simulink model "ieee80211n"  (Simulink 6.0)
settings: Solver=VariableStepDiscrete  StartTime=0.0  StopTime=inf  RelTol=1e-3
PreLoadFcn:
  | load IEEE80211n_init;
values from neighbouring files (symbols this model uses):
  params =     [IEEE80211n_init.mat]    (also in IEEE80211n_settings.m = p)
undefined symbols (not defined in the file or in its folder): magnitude
libraries: commblkintrlv2 x196, dspsigops x143, simulink x136, commdigbbndam2 x98, dspmtrx3 x96, dspsigattribs x69, dspstat3 x38, commutil2 x32, commsequence2 x26, commcnvcod2 x10, dspindex x9, dspmlti3 x8
(part 2 of 12)

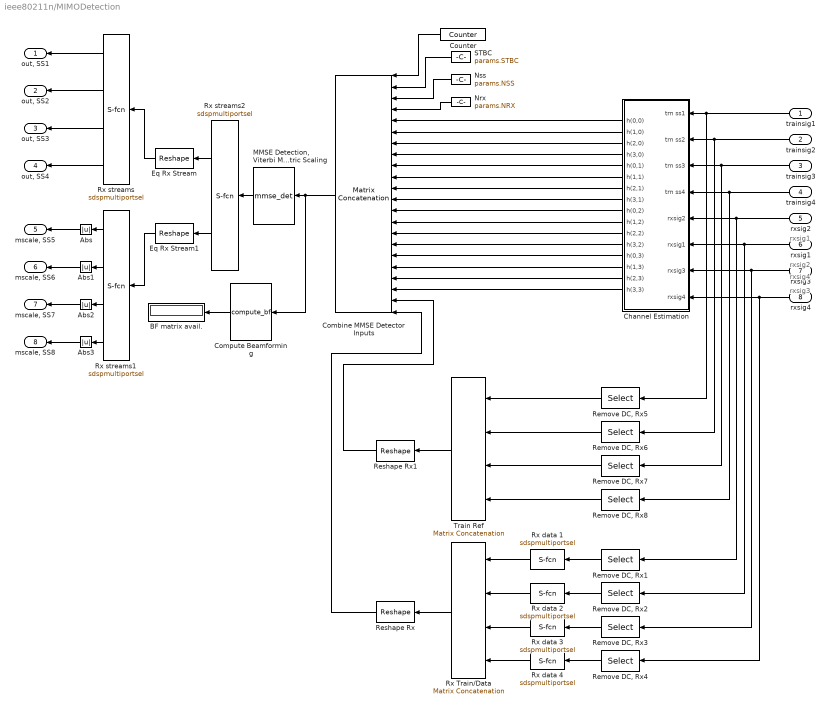
== system ieee80211n/MIMODetection ==
  note: rxsig1
  note: rxsig2
  note: rxsig3
  note: rxsig4
  trainsig1 : Inport  Orientation=left  Port=1  LatchInput=off
  trainsig2 : Inport  Orientation=left  Port=2  LatchInput=off
  trainsig3 : Inport  Orientation=left  Port=3  LatchInput=off
  trainsig4 : Inport  Orientation=left  Port=4  LatchInput=off
  rxsig2 : Inport  Orientation=left  Port=5  LatchInput=off
  rxsig1 : Inport  Orientation=left  Port=6  LatchInput=off
  rxsig3 : Inport  Orientation=left  Port=7  LatchInput=off
  rxsig4 : Inport  Orientation=left  Port=8  LatchInput=off
  Abs{,1..3} (4 alike) : Abs  Orientation=left
  BF matrix avail. : Display
  Channel Estimation : Subsystem  Orientation=left
  Combine MMSE Detector Inputs : simulink/Math Operations/Matrix Concatenation  Orientation=left  numInports=22  catMethod=Vertical
  Compute Beamforming : MATLABFcn  Orientation=left  MATLABFcn=compute_bf  OutputDimensions=[1 1]  Output1D=off
  Counter : dspswit3/Counter  Orientation=left  Direction=Up  CountEvent=Free running  CounterSize=32 bits  MaxCount=255  InitialCount=0  Output=Count  HitValue=32  ResetInput=off  SamplesPerFrame=1  Ts=params.minBitPeriod*(params.NSS*params.maxBitsPerBlock)  CntDtype=double  HitDtype=Logical
  Eq Rx Stream : simulink/Math Operations/Reshape  Orientation=left  OutputDimensionality=Customize  OutputDimensions=[4*56, params.OFDMSymPerFrame]
  Eq Rx Stream1 : simulink/Math Operations/Reshape  Orientation=left  OutputDimensionality=Customize  OutputDimensions=[4*56, params.OFDMSymPerFrame]
  "MMSE Detection, Viterbi Metric Scaling" : MATLABFcn  Orientation=left  MATLABFcn=mmse_det  OutputDimensions=[2*4*56*params.OFDMSymPerFrame 1]  Output1D=off
  Nrx : Constant  Orientation=left  Value=params.NRX
  Nss : Constant  Orientation=left  Value=params.NSS
  Remove DC, Rx{1..8} (8 alike) : Selector  Orientation=left  InputType=Matrix  Elements=[1 3]  Rows=[1:28 30:57]  Columns=-1  InputPortWidth=3
  Reshape Rx : simulink/Math Operations/Reshape  Orientation=left  OutputDimensionality=Customize  OutputDimensions=[4*56*(params.OFDMSymPerFrame+params.OFDM_HTLTF_SymPerFrame),1]
  Reshape Rx1 : simulink/Math Operations/Reshape  Orientation=left  OutputDimensionality=Customize  OutputDimensions=[4*56*(params.OFDM_HTLTF_SymPerFrame),1]
  Rx Train/Data : simulink/Math Operations/Matrix Concatenation  Orientation=left  numInports=4  catMethod=Vertical
  Rx data 1 : S-Function  Orientation=left  AncestorBlock=dspindex/Multiport Selector  FunctionName=sdspmultiportsel  Parameters=rowsOrCols, numOutports, flatIdxVect, flatLenVect, idxErrMode  mask(Multiport Selector){rowsOrCols=Columns, idxCellArray={(params.OFDM_TotPreamblePerFrame-params.OFDM_HTLTF_SymPerFrame+1) :params.OFDMTotSymPerFrame}, idxErrMode=Clip Index}
      mask prompts: rowsOrCols "Select:"; idxCellArray "Indices to output:"; idxErrMode "Invalid index:"
      mask help: Output specified rows or columns to one or more output ports. The number of output ports is determined by the number of index vectors, each specified as a separate vector entry in a cell array. Indices are 1-based and need not be unique.
      mask init:
      | [numOutports, flatLenVect, flatIdxVect] = dspblkmultiportsel(idxCellArray);
      mask Help: web(dspbhelp);
      mask StyleString: popup(Rows|Columns),edit,popup(Clip Index|Clip and Warn|Generate Error)
      mask Display: disp(['Select\n' &1]);
  Rx data 2 : S-Function  Orientation=left  AncestorBlock=dspindex/Multiport Selector  FunctionName=sdspmultiportsel  Parameters=rowsOrCols, numOutports, flatIdxVect, flatLenVect, idxErrMode  mask(Multiport Selector){rowsOrCols=Columns, idxCellArray={(params.OFDM_TotPreamblePerFrame-params.OFDM_HTLTF_SymPerFrame+1) :params.OFDMTotSymPerFrame}, idxErrMode=Clip Index}
      mask prompts: rowsOrCols "Select:"; idxCellArray "Indices to output:"; idxErrMode "Invalid index:"
      mask help: Output specified rows or columns to one or more output ports. The number of output ports is determined by the number of index vectors, each specified as a separate vector entry in a cell array. Indices are 1-based and need not be unique.
      mask init:
      | [numOutports, flatLenVect, flatIdxVect] = dspblkmultiportsel(idxCellArray);
      mask Help: web(dspbhelp);
      mask StyleString: popup(Rows|Columns),edit,popup(Clip Index|Clip and Warn|Generate Error)
      mask Display: disp(['Select\n' &1]);
  Rx data 3 : S-Function  Orientation=left  AncestorBlock=dspindex/Multiport Selector  FunctionName=sdspmultiportsel  Parameters=rowsOrCols, numOutports, flatIdxVect, flatLenVect, idxErrMode  mask(Multiport Selector){rowsOrCols=Columns, idxCellArray={(params.OFDM_TotPreamblePerFrame-params.OFDM_HTLTF_SymPerFrame+1) :params.OFDMTotSymPerFrame}, idxErrMode=Clip Index}
      mask prompts: rowsOrCols "Select:"; idxCellArray "Indices to output:"; idxErrMode "Invalid index:"
      mask help: Output specified rows or columns to one or more output ports. The number of output ports is determined by the number of index vectors, each specified as a separate vector entry in a cell array. Indices are 1-based and need not be unique.
      mask init:
      | [numOutports, flatLenVect, flatIdxVect] = dspblkmultiportsel(idxCellArray);
      mask Help: web(dspbhelp);
      mask StyleString: popup(Rows|Columns),edit,popup(Clip Index|Clip and Warn|Generate Error)
      mask Display: disp(['Select\n' &1]);
  Rx data 4 : S-Function  Orientation=left  AncestorBlock=dspindex/Multiport Selector  FunctionName=sdspmultiportsel  Parameters=rowsOrCols, numOutports, flatIdxVect, flatLenVect, idxErrMode  mask(Multiport Selector){rowsOrCols=Columns, idxCellArray={(params.OFDM_TotPreamblePerFrame-params.OFDM_HTLTF_SymPerFrame+1) :params.OFDMTotSymPerFrame}, idxErrMode=Clip Index}
      mask prompts: rowsOrCols "Select:"; idxCellArray "Indices to output:"; idxErrMode "Invalid index:"
      mask help: Output specified rows or columns to one or more output ports. The number of output ports is determined by the number of index vectors, each specified as a separate vector entry in a cell array. Indices are 1-based and need not be unique.
      mask init:
      | [numOutports, flatLenVect, flatIdxVect] = dspblkmultiportsel(idxCellArray);
      mask Help: web(dspbhelp);
      mask StyleString: popup(Rows|Columns),edit,popup(Clip Index|Clip and Warn|Generate Error)
      mask Display: disp(['Select\n' &1]);
  Rx streams : S-Function  Orientation=left  AncestorBlock=dspindex/Multiport Selector  FunctionName=sdspmultiportsel  Parameters=rowsOrCols, numOutports, flatIdxVect, flatLenVect, idxErrMode  mask(Multiport Selector){rowsOrCols=Rows, idxCellArray={1:56  1*56+(1:56)  2*56+(1:56)  3*56+(1:56)}, idxErrMode=Clip Index}
      mask prompts: rowsOrCols "Select:"; idxCellArray "Indices to output:"; idxErrMode "Invalid index:"
      mask help: Output specified rows or columns to one or more output ports. The number of output ports is determined by the number of index vectors, each specified as a separate vector entry in a cell array. Indices are 1-based and need not be unique.
      mask init:
      | [numOutports, flatLenVect, flatIdxVect] = dspblkmultiportsel(idxCellArray);
      mask Help: web(dspbhelp);
      mask StyleString: popup(Rows|Columns),edit,popup(Clip Index|Clip and Warn|Generate Error)
      mask Display: disp(['Select\n' &1]);
  Rx streams1 : S-Function  Orientation=left  AncestorBlock=dspindex/Multiport Selector  FunctionName=sdspmultiportsel  Parameters=rowsOrCols, numOutports, flatIdxVect, flatLenVect, idxErrMode  mask(Multiport Selector){rowsOrCols=Rows, idxCellArray={1:56  1*56+(1:56)  2*56+(1:56)  3*56+(1:56)}, idxErrMode=Clip Index}
      mask prompts: rowsOrCols "Select:"; idxCellArray "Indices to output:"; idxErrMode "Invalid index:"
      mask help: Output specified rows or columns to one or more output ports. The number of output ports is determined by the number of index vectors, each specified as a separate vector entry in a cell array. Indices are 1-based and need not be unique.
      mask init:
      | [numOutports, flatLenVect, flatIdxVect] = dspblkmultiportsel(idxCellArray);
      mask Help: web(dspbhelp);
      mask StyleString: popup(Rows|Columns),edit,popup(Clip Index|Clip and Warn|Generate Error)
      mask Display: disp(['Select\n' &1]);
  Rx streams2 : S-Function  Orientation=left  AncestorBlock=dspindex/Multiport Selector  FunctionName=sdspmultiportsel  Parameters=rowsOrCols, numOutports, flatIdxVect, flatLenVect, idxErrMode  mask(Multiport Selector){rowsOrCols=Rows, idxCellArray={(1:4*56*params.OFDMSymPerFrame) 4*56*params.OFDMSymPerFrame+(1:4*56*params.OFDMSymPerFrame)}, idxErrMode=Clip Index}
      mask prompts: rowsOrCols "Select:"; idxCellArray "Indices to output:"; idxErrMode "Invalid index:"
      mask help: Output specified rows or columns to one or more output ports. The number of output ports is determined by the number of index vectors, each specified as a separate vector entry in a cell array. Indices are 1-based and need not be unique.
      mask init:
      | [numOutports, flatLenVect, flatIdxVect] = dspblkmultiportsel(idxCellArray);
      mask Help: web(dspbhelp);
      mask StyleString: popup(Rows|Columns),edit,popup(Clip Index|Clip and Warn|Generate Error)
      mask Display: disp(['Select\n' &1]);
  STBC : Constant  Orientation=left  Value=params.STBC  VectorParams1D=off
  Train Ref : simulink/Math Operations/Matrix Concatenation  Orientation=left  numInports=4  catMethod=Vertical
  "out, SS1" : Outport  Orientation=left
  "out, SS2" : Outport  Orientation=left  Port=2
  "out, SS3" : Outport  Orientation=left  Port=3
  "out, SS4" : Outport  Orientation=left  Port=4
  "mscale, SS5" : Outport  Orientation=left  Port=5
  "mscale, SS6" : Outport  Orientation=left  Port=6
  "mscale, SS7" : Outport  Orientation=left  Port=7
  "mscale, SS8" : Outport  Orientation=left  Port=8
  wires:
  trainsig1/1 -> Channel Estimation/1(trn ss1), "Remove DC, Rx5"/1
  trainsig2/1 -> Channel Estimation/2(trn ss2), "Remove DC, Rx6"/1
  trainsig3/1 -> Channel Estimation/3(trn ss3), "Remove DC, Rx7"/1
  trainsig4/1 -> Channel Estimation/4(trn ss4), "Remove DC, Rx8"/1
  rxsig2/1 -> Channel Estimation/5(rxsig2), "Remove DC, Rx1"/1
  rxsig1/1 -> Channel Estimation/6(rxsig1), "Remove DC, Rx2"/1
  rxsig3/1 -> Channel Estimation/7(rxsig3), "Remove DC, Rx3"/1
  rxsig4/1 -> Channel Estimation/8(rxsig4), "Remove DC, Rx4"/1
  Channel Estimation/1(h(0,0)) -> Combine MMSE Detector Inputs/5
  Channel Estimation/2(h(1,0)) -> Combine MMSE Detector Inputs/6
  Channel Estimation/3(h(2,0)) -> Combine MMSE Detector Inputs/7
  Channel Estimation/4(h(3,0)) -> Combine MMSE Detector Inputs/8
  Channel Estimation/5(h(0,1)) -> Combine MMSE Detector Inputs/9
  Channel Estimation/6(h(1,1)) -> Combine MMSE Detector Inputs/10
  Channel Estimation/7(h(2,1)) -> Combine MMSE Detector Inputs/11
  Channel Estimation/8(h(3,1)) -> Combine MMSE Detector Inputs/12
  Channel Estimation/9(h(0,2)) -> Combine MMSE Detector Inputs/13
  Channel Estimation/10(h(1,2)) -> Combine MMSE Detector Inputs/14
  Channel Estimation/11(h(2,2)) -> Combine MMSE Detector Inputs/15
  Channel Estimation/12(h(3,2)) -> Combine MMSE Detector Inputs/16
  Channel Estimation/13(h(0,3)) -> Combine MMSE Detector Inputs/17
  Channel Estimation/14(h(1,3)) -> Combine MMSE Detector Inputs/18
  Channel Estimation/15(h(2,3)) -> Combine MMSE Detector Inputs/19
  Channel Estimation/16(h(3,3)) -> Combine MMSE Detector Inputs/20
  Combine MMSE Detector Inputs/1 -> Compute Beamforming/1, "MMSE Detection, Viterbi Metric Scaling"/1
  "Remove DC, Rx1"/1 -> Rx data 1/1
  "Remove DC, Rx2"/1 -> Rx data 2/1
  "Remove DC, Rx3"/1 -> Rx data 3/1
  "Remove DC, Rx4"/1 -> Rx data 4/1
  Eq Rx Stream/1 -> Rx streams/1
  Rx streams/1 -> "out, SS1"/1
  Rx streams/2 -> "out, SS2"/1
  Rx streams/3 -> "out, SS3"/1
  Rx streams/4 -> "out, SS4"/1
  Rx data 1/1 -> Rx Train/Data/1
  Rx data 2/1 -> Rx Train/Data/2
  Rx data 3/1 -> Rx Train/Data/3
  Rx data 4/1 -> Rx Train/Data/4
  Rx Train/Data/1 -> Reshape Rx/1
  Reshape Rx/1 -> Combine MMSE Detector Inputs/22
  Nss/1 -> Combine MMSE Detector Inputs/3
  "Remove DC, Rx8"/1 -> Train Ref/4
  "Remove DC, Rx7"/1 -> Train Ref/3
  "Remove DC, Rx6"/1 -> Train Ref/2
  "Remove DC, Rx5"/1 -> Train Ref/1
  Train Ref/1 -> Reshape Rx1/1
  Reshape Rx1/1 -> Combine MMSE Detector Inputs/21
  Nrx/1 -> Combine MMSE Detector Inputs/4
  STBC/1 -> Combine MMSE Detector Inputs/2
  Counter/1 -> Combine MMSE Detector Inputs/1
  Compute Beamforming/1 -> BF matrix avail./1
  Rx streams1/1 -> Abs/1
  Rx streams1/2 -> Abs1/1
  Rx streams1/3 -> Abs2/1
  Rx streams1/4 -> Abs3/1
  Abs/1 -> "mscale, SS5"/1
  Abs1/1 -> "mscale, SS6"/1
  Abs2/1 -> "mscale, SS7"/1
  Abs3/1 -> "mscale, SS8"/1
  "MMSE Detection, Viterbi Metric Scaling"/1 -> Rx streams2/1
  Rx streams2/1 -> Eq Rx Stream/1
  Rx streams2/2 -> Eq Rx Stream1/1
  Eq Rx Stream1/1 -> Rx streams1/1

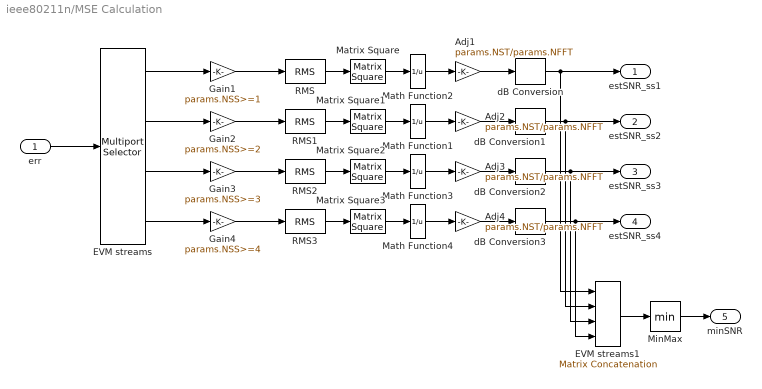
== system ieee80211n/MSE Calculation ==
  err : Inport  Port=1  LatchInput=off
  Adj{1..4} (4 alike) : Gain  Gain=params.NST/params.NFFT  SaturateOnIntegerOverflow=on
  EVM streams : dspindex/Multiport Selector  rowsOrCols=Columns  idxCellArray={1, 2, 3, 4}  idxErrMode=Clip Index
  EVM streams1 : simulink/Math Operations/Matrix Concatenation  numInports=4  catMethod=Horizontal
  Gain1 : Gain  Gain=params.NSS>=1  SaturateOnIntegerOverflow=on
  Gain2 : Gain  Gain=params.NSS>=2  SaturateOnIntegerOverflow=on
  Gain3 : Gain  Gain=params.NSS>=3  SaturateOnIntegerOverflow=on
  Gain4 : Gain  Gain=params.NSS>=4  SaturateOnIntegerOverflow=on
  Math Function{1..4} (4 alike) : Math  Operator=reciprocal  SaturateOnIntegerOverflow=on
  Matrix Square{,1..3} (4 alike) : dspmtrx3/Matrix Square
  MinMax : MinMax  SaturateOnIntegerOverflow=on  InputSameDT=on
  RMS{,1..3} (4 alike) : dspstat3/RMS  run=off  reset_popup=None
  dB Conversion{,1..3} (4 alike) : dspmathops/dB Conversion  dBtype=dB  intype=Power  R=1  fuzz=on
  estSNR_ss1 : Outport
  estSNR_ss2 : Outport  Port=2
  estSNR_ss3 : Outport  Port=3
  estSNR_ss4 : Outport  Port=4
  minSNR : Outport  Port=5
  wires:
  Matrix Square/1 -> Math Function2/1
  Math Function2/1 -> Adj1/1
  RMS/1 -> Matrix Square/1
  err/1 -> EVM streams/1
  dB Conversion/1 -> estSNR_ss1/1, EVM streams1/1
  Matrix Square1/1 -> Math Function1/1
  Math Function1/1 -> Adj2/1
  RMS1/1 -> Matrix Square1/1
  Matrix Square2/1 -> Math Function3/1
  Math Function3/1 -> Adj3/1
  RMS2/1 -> Matrix Square2/1
  Matrix Square3/1 -> Math Function4/1
  Math Function4/1 -> Adj4/1
  RMS3/1 -> Matrix Square3/1
  dB Conversion1/1 -> estSNR_ss2/1, EVM streams1/2
  dB Conversion2/1 -> estSNR_ss3/1, EVM streams1/3
  dB Conversion3/1 -> estSNR_ss4/1, EVM streams1/4
  EVM streams/1 -> Gain1/1
  EVM streams/2 -> Gain2/1
  EVM streams/3 -> Gain3/1
  EVM streams/4 -> Gain4/1
  EVM streams1/1 -> MinMax/1
  MinMax/1 -> minSNR/1
  Gain1/1 -> RMS/1
  Gain2/1 -> RMS1/1
  Gain3/1 -> RMS2/1
  Gain4/1 -> RMS3/1
  Adj1/1 -> dB Conversion/1
  Adj2/1 -> dB Conversion1/1
  Adj3/1 -> dB Conversion2/1
  Adj4/1 -> dB Conversion3/1

== system ieee80211n/ModulatorBank ==
  mode : Inport  Port=1  LatchInput=off
  txbits : Inport  Port=2  LatchInput=off
  CC_PuncBank : Subsystem  mask(IEEE 802.11a modulator-coder bank.){}
      mask init:
      | code = {'1/2' '1/2' '3/4' '1/2' '3/4' '2/3' '3/4' '5/6'};
      | 
      | % modulation-specific
      | TS1 = 'poly2trellis(7, [171 133])';
      | TS2 = 'poly2trellis(7, [133 171])';
      | trellisStructure = {TS1 TS1 TS1 TS1 TS1 TS2 TS2 TS2};
      | 
      | % code-specific
      | PV = {'[1]', '[1 1 1 0].''', '[1 1 1 0 0 1].''', '[1]', '[1 1 1 0 0 1 1 0 0 1].'''};
      | punctureVector = {PV{1} PV{1} PV{3} PV{1} PV{3} PV{2} PV{3} PV{5}};
      | 
      | if 0
      |   for n = 1:numModulators
      |     blk = [gcb '/Modulator ' num2str(n)];
      |     set_param(blk, 'numSymbols', num2str(nSymbolsPerFrame));
      |     set_param(blk, 'modulation', modulation{n});
      |     set_param(blk, 'code', code{n});
      |     set_param(blk, 'trellisStructure', trellisStructure{n});
      |     set_param(blk, 'punctureVector', punctureVector{n});
      |   end
      | end
      mask Display: disp('Conv. Coding +\n Puncturing')
  Group into OFDM symbols : Subsystem
      mask Display: disp('OFDM\nSymbols\nSS1')
  Group into OFDM symbols1 : Subsystem
      mask Display: disp('OFDM\nSymbols\nSS2')
  Group into OFDM symbols2 : Subsystem
      mask Display: disp('OFDM\nSymbols\nSS3')
  Group into OFDM symbols3 : Subsystem
      mask Display: disp('OFDM\nSymbols\nSS4')
  ModulatorSS1 : Subsystem  mask(IEEE 802.11n modulator-coder bank.){nSymbolsPerFrame=params.numTxSymbols}
      mask prompts: nSymbolsPerFrame "Number of symbols per frame:"
      mask init:
      | numModulators = 8;
      | modulation = {'BPSK' 'QPSK' 'QPSK' '16-QAM' '16-QAM' '64-QAM' '64-QAM' '64-QAM'};
      | code = {'1/2' '1/2' '3/4' '1/2' '3/4' '2/3' '3/4' '5/6'};
      | 
      | % modulation-specific
      | TS1 = 'poly2trellis(7, [171 133])';
      | TS2 = 'poly2trellis(7, [133 171])';
      | trellisStructure = {TS1 TS1 TS1 TS1 TS1 TS2 TS2 TS2};
      | 
      | % code-specific
      | PV = {'[1]', '[1 1 1 0].''', '[1 1 1 0 0 1].''', '[1]', '[1 1 1 0 0 1 1 0 0 1].'''};
      | punctureVector = {PV{1} PV{1} PV{3} PV{1} PV{3} PV{2} PV{3} PV{5}};
      | 
      | for n = 1:numModulators
      |     blk = [gcb '/Modulator ' num2str(n)];
      |     set_param(blk, 'numSymbols', num2str(nSymbolsPerFrame));
      |     set_param(blk, 'modulation', modulation{n});
      |     set_param(blk, 'code', code{n});
      |     set_param(blk, 'trellisStructure', trellisStructure{n});
      |     set_param(blk, 'punctureVector', punctureVector{n});
      | end
      mask Display: disp('Modulator\nBank\nSS1')
  ModulatorSS2 : Subsystem  mask(IEEE 802.11n modulator-coder bank.){nSymbolsPerFrame=params.numTxSymbols}
      mask prompts: nSymbolsPerFrame "Number of symbols per frame:"
      mask init: same as ieee80211n/ModulatorBank/ModulatorSS1
      mask Display: disp('Modulator\nBank\nSS2')
  ModulatorSS3 : Subsystem  mask(IEEE 802.11n modulator-coder bank.){nSymbolsPerFrame=params.numTxSymbols}
      mask prompts: nSymbolsPerFrame "Number of symbols per frame:"
      mask init:
      | numModulators = 8;
      | modulation = {'BPSK' 'QPSK' 'QPSK' '16-QAM' '16-QAM' '64-QAM' '64-QAM' '64-QAM'};
      | code = {'1/2' '1/2' '3/4' '1/2' '3/4' '2/3' '3/4' '5/6'};
      | 
      | % modulation-specific
      | TS1 = 'poly2trellis(7, [171 133])';
      | TS2 = 'poly2trellis(7, [133 171])';
      | trellisStructure = {TS1 TS1 TS1 TS1 TS1 TS2 TS2 TS2};
      | 
      | % code-specific
      | PV = {'[1]', '[1 1 1 0].''', '[1 1 1 0 0 1].''', '[1]', '[1 1 1 0 0 1 1 0 0 1].'''};
      | punctureVector = {PV{1} PV{1} PV{3} PV{1} PV{3} PV{2} PV{3} PV{5}};
      | 
      | for n = 1:numModulators
      |     blk = [gcb '/Modulator ' num2str(n)];
      |     set_param(blk, 'numSymbols', num2str(nSymbolsPerFrame));
      |     set_param(blk, 'modulation', modulation{n});
      |     set_param(blk, 'code', code{n});
      |     set_param(blk, 'trellisStructure', trellisStructure{n});
      |     set_param(blk, 'punctureVector', punctureVector{n});
      | end
      mask Display: disp('Modulator\nBank\nSS3')
  ModulatorSS4 : Subsystem  mask(IEEE 802.11n modulator-coder bank.){nSymbolsPerFrame=params.numTxSymbols}
      mask prompts: nSymbolsPerFrame "Number of symbols per frame:"
      mask init: same as ieee80211n/ModulatorBank/ModulatorSS1
      mask Display: disp('Modulator\nBank\nSS4')
  Nss : Constant  Value=params.NSS
  Parsing Input : simulink/Math Operations/Matrix Concatenation  numInports=4  catMethod=Vertical
  Spatial Parsing : MATLABFcn  MATLABFcn=spatial_parse  OutputDimensions=[4*params.maxTxBitsPerBlock 1]  Output1D=off
  Spatial Streams : S-Function  AncestorBlock=dspindex/Multiport Selector  FunctionName=sdspmultiportsel  Parameters=rowsOrCols, numOutports, flatIdxVect, flatLenVect, idxErrMode  mask(Multiport Selector){rowsOrCols=Rows, idxCellArray={1:params.maxTxBitsPerBlock  (params.maxTxBitsPerBlock+1):(2*params.maxTxBitsPerBlock)  (2*params.maxTxBitsPerBlock+1):(3*params.maxTxBitsPerBlock)  (3*params.maxTxBitsPerBlock+1):(4*params.maxTxBitsPerBlock) }, idxErrMode=Clip Index}
      mask prompts: rowsOrCols "Select:"; idxCellArray "Indices to output:"; idxErrMode "Invalid index:"
      mask help: Output specified rows or columns to one or more output ports. The number of output ports is determined by the number of index vectors, each specified as a separate vector entry in a cell array. Indices are 1-based and need not be unique.
      mask init:
      | [numOutports, flatLenVect, flatIdxVect] = dspblkmultiportsel(idxCellArray);
      mask Help: web(dspbhelp);
      mask StyleString: popup(Rows|Columns),edit,popup(Clip Index|Clip and Warn|Generate Error)
      mask Display: disp(['Select\n' &1]);
  blksize : Constant  Value=params.maxTxBitsPerBlock
  "out, SS1" : Outport
  "out, SS2" : Outport  Port=2
  "out, SS3" : Outport  Port=3
  "out, SS4" : Outport  Port=4
  wires:
  mode/1 -> CC_PuncBank/1(mode), ModulatorSS2/1(mode), ModulatorSS3/1(mode), ModulatorSS4/1(mode), ModulatorSS1/1(mode), Parsing Input/1
  ModulatorSS1/1(sig) -> Group into OFDM symbols/1(in)
  Group into OFDM symbols/1(out) -> "out, SS1"/1
  ModulatorSS2/1(sig) -> Group into OFDM symbols1/1(in)
  Group into OFDM symbols1/1(out) -> "out, SS2"/1
  ModulatorSS3/1(sig) -> Group into OFDM symbols2/1(in)
  Group into OFDM symbols2/1(out) -> "out, SS3"/1
  ModulatorSS4/1(sig) -> Group into OFDM symbols3/1(in)
  Group into OFDM symbols3/1(out) -> "out, SS4"/1
  txbits/1 -> CC_PuncBank/2(txbits)
  Parsing Input/1 -> Spatial Parsing/1
  CC_PuncBank/1(sig) -> Parsing Input/4
  Spatial Parsing/1 -> Spatial Streams/1
  Spatial Streams/1 -> ModulatorSS1/2(txbits)
  Spatial Streams/2 -> ModulatorSS2/2(txbits)
  Spatial Streams/3 -> ModulatorSS3/2(txbits)
  Spatial Streams/4 -> ModulatorSS4/2(txbits)
  Nss/1 -> Parsing Input/2
  blksize/1 -> Parsing Input/3

== system ieee80211n/Multiplex ==
  In1 : Inport  Port=1  LatchInput=off
  Reshape2 : simulink/Math Operations/Reshape  OutputDimensionality=Column vector  OutputDimensions=1600
  Out1 : Outport
  wires:
  In1/1 -> Reshape2/1
  Reshape2/1 -> Out1/1

== system ieee80211n/Multiplex1 ==
  In1 : Inport  Port=1  LatchInput=off
  Reshape2 : simulink/Math Operations/Reshape  OutputDimensionality=Column vector  OutputDimensions=1600
  Out1 : Outport
  wires:
  In1/1 -> Reshape2/1
  Reshape2/1 -> Out1/1

== system ieee80211n/Multiplex2 ==
  In1 : Inport  Port=1  LatchInput=off
  Reshape2 : simulink/Math Operations/Reshape  OutputDimensionality=Column vector  OutputDimensions=1600
  Out1 : Outport
  wires:
  In1/1 -> Reshape2/1
  Reshape2/1 -> Out1/1

== system ieee80211n/Multiplex3 ==
  In1 : Inport  Port=1  LatchInput=off
  Reshape2 : simulink/Math Operations/Reshape  OutputDimensionality=Column vector  OutputDimensions=1600
  Out1 : Outport
  wires:
  In1/1 -> Reshape2/1
  Reshape2/1 -> Out1/1

== system ieee80211n/PER Curve ==
  mode : Inport  Port=1  LatchInput=off
  txbits : Inport  Port=2  LatchInput=off
  rxbits : Inport  Port=3  LatchInput=off
  Counter : dspswit3/Counter  Direction=Up  CountEvent=Free running  CounterSize=32 bits  MaxCount=255  InitialCount=0  Output=Count  HitValue=32  ResetInput=off  SamplesPerFrame=1  Ts=params.minBitPeriod*(params.NSS*params.maxBitsPerBlock)  CntDtype=double  HitDtype=Logical
  PER graph data : simulink/Math Operations/Matrix Concatenation  numInports=5  catMethod=Vertical
  Plot PER graph : MATLABFcn  MATLABFcn=per_graph  OutputDimensions=[1 1]  Output1D=off
  Reshape : simulink/Math Operations/Reshape  OutputDimensionality=Column vector  OutputDimensions=[1,1]
  Reshape1 : simulink/Math Operations/Reshape  OutputDimensionality=Column vector  OutputDimensions=[1,1]
  Reshape2 : simulink/Math Operations/Reshape  OutputDimensionality=Column vector  OutputDimensions=[1,1]
  blksize : Constant  Value=params.NSS*params.bitsPerBlock  VectorParams1D=off
  out : Outport
  wires:
  Plot PER graph/1 -> out/1
  PER graph data/1 -> Plot PER graph/1
  blksize/1 -> Reshape2/1
  mode/1 -> PER graph data/3
  txbits/1 -> Reshape1/1
  rxbits/1 -> Reshape/1
  Counter/1 -> PER graph data/1
  Reshape/1 -> PER graph data/5
  Reshape1/1 -> PER graph data/4
  Reshape2/1 -> PER graph data/2

== system ieee80211n/PER calculation ==
  tx : Inport  Port=1  LatchInput=off
  mode : Inport  Port=2  LatchInput=off
  rx : Inport  Port=3  LatchInput=off
  Bit indices : Subsystem
  Error Rate Calculation : commsink2/Error Rate Calculation  N=0  st_delay=0  cp_mode=Select samples from port  subframe=[]  PMode=Port  WsName=ErrorVec  RsMode2=off  stop=off  numErr=100  maxBits=1e6
  Selector : Selector  Elements=2  InputPortWidth=3
  Translate to packet error rate : Subsystem
  Variable Integer Delay : S-Function  AncestorBlock=dspsigops/Variable Integer Delay  FunctionName=sdspvidly2  Parameters=dmax,ic  mask(Variable Integer Delay){dmax=200, ic=0}
      mask prompts: dmax "Maximum delay (samples):"; ic "Initial conditions:"
      mask help: Delay discrete-time input by a time-varying integer number of sample periods specified by the "delay" input.
      settings: CopyFcn=dspfixptcopycallback
      mask Help: web(dspbhelp);
      mask Display:
      | text(0.5,0.4,'z','horiz','right')
      | text(0.5,0.6,'-i','horiz','left')
      | port_label('input',1,'In')
      | port_label('input',2,'Delay')
      | port_label('output',1,'Out')
  link delay : IEEE80211a_lib/Select value  vector=params.link_delay.'
  PER : Outport
  wires:
  rx/1 -> Error Rate Calculation/2
  link delay/1 -> Bit indices/2(delay), Variable Integer Delay/2
  Selector/1 -> Translate to packet error rate/1(bit errors)
  Translate to packet error rate/1(PER) -> PER/1
  Variable Integer Delay/1 -> Error Rate Calculation/1
  Bit indices/1(sel) -> Error Rate Calculation/3
  mode/1 -> Bit indices/1(mode), link delay/1
  Error Rate Calculation/1 -> Selector/1
  tx/1 -> Variable Integer Delay/1

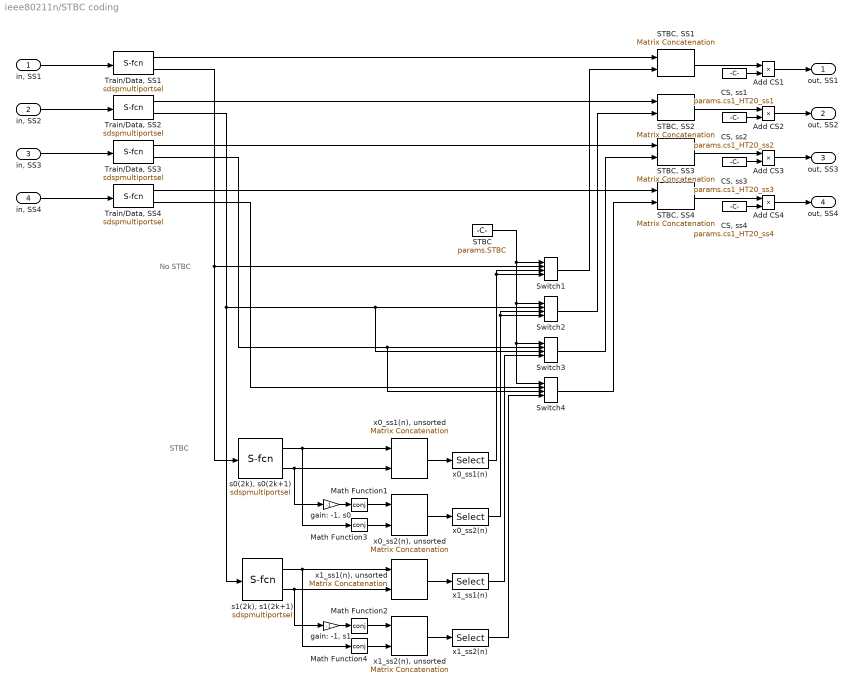
== system ieee80211n/STBC coding ==
  note: No STBC
  note: STBC
  "in, SS1" : Inport  Port=1  LatchInput=off
  "in, SS2" : Inport  Port=2  LatchInput=off
  "in, SS3" : Inport  Port=3  LatchInput=off
  "in, SS4" : Inport  Port=4  LatchInput=off
  Add CS{1..4} (4 alike) : Product  Inputs=**  SaturateOnIntegerOverflow=on
  "CS, ss1" : Constant  Value=params.cs1_HT20_ss1  VectorParams1D=off
  "CS, ss2" : Constant  Value=params.cs1_HT20_ss2  VectorParams1D=off
  "CS, ss3" : Constant  Value=params.cs1_HT20_ss3  VectorParams1D=off
  "CS, ss4" : Constant  Value=params.cs1_HT20_ss4  VectorParams1D=off
  Math Function{1..4} (4 alike) : Math  Operator=conj  SaturateOnIntegerOverflow=on
  STBC : Constant  Value=params.STBC
  STBC, SS{1..4} (4 alike) : simulink/Math Operations/Matrix Concatenation  numInports=2  catMethod=Horizontal
  Switch{1..4} (4 alike) : MultiPortSwitch  Inputs=3  zeroidx=on  SaturateOnIntegerOverflow=on
  "Train/Data, SS1" : S-Function  AncestorBlock=dspindex/Multiport Selector  FunctionName=sdspmultiportsel  Parameters=rowsOrCols, numOutports, flatIdxVect, flatLenVect, idxErrMode  mask(Multiport Selector){rowsOrCols=Columns, idxCellArray={params.OFDM_PreambleIndices,params.OFDM_DatamodeIndices}, idxErrMode=Clip Index}
      mask prompts: rowsOrCols "Select:"; idxCellArray "Indices to output:"; idxErrMode "Invalid index:"
      mask help: Output specified rows or columns to one or more output ports. The number of output ports is determined by the number of index vectors, each specified as a separate vector entry in a cell array. Indices are 1-based and need not be unique.
      mask init:
      | [numOutports, flatLenVect, flatIdxVect] = dspblkmultiportsel(idxCellArray);
      mask Help: web(dspbhelp);
      mask StyleString: popup(Rows|Columns),edit,popup(Clip Index|Clip and Warn|Generate Error)
      mask Display: disp(['Select\n' &1]);
  "Train/Data, SS2" : S-Function  AncestorBlock=dspindex/Multiport Selector  FunctionName=sdspmultiportsel  Parameters=rowsOrCols, numOutports, flatIdxVect, flatLenVect, idxErrMode  mask(Multiport Selector){rowsOrCols=Columns, idxCellArray={params.OFDM_PreambleIndices,params.OFDM_DatamodeIndices}, idxErrMode=Clip Index}
      mask prompts: rowsOrCols "Select:"; idxCellArray "Indices to output:"; idxErrMode "Invalid index:"
      mask help: Output specified rows or columns to one or more output ports. The number of output ports is determined by the number of index vectors, each specified as a separate vector entry in a cell array. Indices are 1-based and need not be unique.
      mask init:
      | [numOutports, flatLenVect, flatIdxVect] = dspblkmultiportsel(idxCellArray);
      mask Help: web(dspbhelp);
      mask StyleString: popup(Rows|Columns),edit,popup(Clip Index|Clip and Warn|Generate Error)
      mask Display: disp(['Select\n' &1]);
  "Train/Data, SS3" : S-Function  AncestorBlock=dspindex/Multiport Selector  FunctionName=sdspmultiportsel  Parameters=rowsOrCols, numOutports, flatIdxVect, flatLenVect, idxErrMode  mask(Multiport Selector){rowsOrCols=Columns, idxCellArray={params.OFDM_PreambleIndices,params.OFDM_DatamodeIndices}, idxErrMode=Clip Index}
      mask prompts: rowsOrCols "Select:"; idxCellArray "Indices to output:"; idxErrMode "Invalid index:"
      mask help: Output specified rows or columns to one or more output ports. The number of output ports is determined by the number of index vectors, each specified as a separate vector entry in a cell array. Indices are 1-based and need not be unique.
      mask init:
      | [numOutports, flatLenVect, flatIdxVect] = dspblkmultiportsel(idxCellArray);
      mask Help: web(dspbhelp);
      mask StyleString: popup(Rows|Columns),edit,popup(Clip Index|Clip and Warn|Generate Error)
      mask Display: disp(['Select\n' &1]);
  "Train/Data, SS4" : S-Function  AncestorBlock=dspindex/Multiport Selector  FunctionName=sdspmultiportsel  Parameters=rowsOrCols, numOutports, flatIdxVect, flatLenVect, idxErrMode  mask(Multiport Selector){rowsOrCols=Columns, idxCellArray={params.OFDM_PreambleIndices,params.OFDM_DatamodeIndices}, idxErrMode=Clip Index}
      mask prompts: rowsOrCols "Select:"; idxCellArray "Indices to output:"; idxErrMode "Invalid index:"
      mask help: Output specified rows or columns to one or more output ports. The number of output ports is determined by the number of index vectors, each specified as a separate vector entry in a cell array. Indices are 1-based and need not be unique.
      mask init:
      | [numOutports, flatLenVect, flatIdxVect] = dspblkmultiportsel(idxCellArray);
      mask Help: web(dspbhelp);
      mask StyleString: popup(Rows|Columns),edit,popup(Clip Index|Clip and Warn|Generate Error)
      mask Display: disp(['Select\n' &1]);
  "gain: -1, s0" : Gain  Gain=-1  SaturateOnIntegerOverflow=on
  "gain: -1, s1" : Gain  Gain=-1  SaturateOnIntegerOverflow=on
  "s0(2k), s0(2k+1)" : S-Function  AncestorBlock=dspindex/Multiport Selector  FunctionName=sdspmultiportsel  Parameters=rowsOrCols, numOutports, flatIdxVect, flatLenVect, idxErrMode  mask(Multiport Selector){rowsOrCols=Columns, idxCellArray={params.TXSTBCInputIndices1, params.TXSTBCInputIndices2}, idxErrMode=Clip Index}
      mask prompts: rowsOrCols "Select:"; idxCellArray "Indices to output:"; idxErrMode "Invalid index:"
      mask help: Output specified rows or columns to one or more output ports. The number of output ports is determined by the number of index vectors, each specified as a separate vector entry in a cell array. Indices are 1-based and need not be unique.
      mask init:
      | [numOutports, flatLenVect, flatIdxVect] = dspblkmultiportsel(idxCellArray);
      mask Help: web(dspbhelp);
      mask StyleString: popup(Rows|Columns),edit,popup(Clip Index|Clip and Warn|Generate Error)
      mask Display: disp(['Select\n' &1]);
  "s1(2k), s1(2k+1)" : S-Function  AncestorBlock=dspindex/Multiport Selector  FunctionName=sdspmultiportsel  Parameters=rowsOrCols, numOutports, flatIdxVect, flatLenVect, idxErrMode  mask(Multiport Selector){rowsOrCols=Columns, idxCellArray={params.TXSTBCInputIndices1, params.TXSTBCInputIndices2}, idxErrMode=Clip Index}
      mask prompts: rowsOrCols "Select:"; idxCellArray "Indices to output:"; idxErrMode "Invalid index:"
      mask help: Output specified rows or columns to one or more output ports. The number of output ports is determined by the number of index vectors, each specified as a separate vector entry in a cell array. Indices are 1-based and need not be unique.
      mask init:
      | [numOutports, flatLenVect, flatIdxVect] = dspblkmultiportsel(idxCellArray);
      mask Help: web(dspbhelp);
      mask StyleString: popup(Rows|Columns),edit,popup(Clip Index|Clip and Warn|Generate Error)
      mask Display: disp(['Select\n' &1]);
  x0_ss1(n) : Selector  InputType=Matrix  Elements=[27:64 1:26]  Rows=-1  Columns=params.TXSTBCShiftIndices  InputPortWidth=64
  "x0_ss1(n), unsorted" : simulink/Math Operations/Matrix Concatenation  numInports=2  catMethod=Horizontal
  x0_ss2(n) : Selector  InputType=Matrix  Elements=[27:64 1:26]  Rows=-1  Columns=params.TXSTBCShiftIndices  InputPortWidth=64
  "x0_ss2(n), unsorted" : simulink/Math Operations/Matrix Concatenation  numInports=2  catMethod=Horizontal
  x1_ss1(n) : Selector  InputType=Matrix  Elements=[27:64 1:26]  Rows=-1  Columns=params.TXSTBCShiftIndices  InputPortWidth=64
  "x1_ss1(n), unsorted" : simulink/Math Operations/Matrix Concatenation  numInports=2  catMethod=Horizontal
  x1_ss2(n) : Selector  InputType=Matrix  Elements=[27:64 1:26]  Rows=-1  Columns=params.TXSTBCShiftIndices  InputPortWidth=64
  "x1_ss2(n), unsorted" : simulink/Math Operations/Matrix Concatenation  numInports=2  catMethod=Horizontal
  "out, SS1" : Outport
  "out, SS2" : Outport  Port=2
  "out, SS3" : Outport  Port=3
  "out, SS4" : Outport  Port=4
  wires:
  "in, SS1"/1 -> "Train/Data, SS1"/1
  "in, SS2"/1 -> "Train/Data, SS2"/1
  "in, SS3"/1 -> "Train/Data, SS3"/1
  "in, SS4"/1 -> "Train/Data, SS4"/1
  "Train/Data, SS1"/1 -> "STBC, SS1"/1
  "Train/Data, SS2"/1 -> "STBC, SS2"/1
  "Train/Data, SS3"/1 -> "STBC, SS3"/1
  "Train/Data, SS4"/1 -> "STBC, SS4"/1
  "Train/Data, SS1"/2 -> "s0(2k), s0(2k+1)"/1, Switch1/2
  "Train/Data, SS2"/2 -> "s1(2k), s1(2k+1)"/1, Switch2/2, Switch3/3
  "Train/Data, SS3"/2 -> Switch3/2, Switch4/3
  "Train/Data, SS4"/2 -> Switch4/2
  STBC/1 -> Switch2/1, Switch3/1, Switch4/1, Switch1/1
  "gain: -1, s0"/1 -> Math Function1/1
  "s0(2k), s0(2k+1)"/2 -> "gain: -1, s0"/1, "x0_ss1(n), unsorted"/2
  "gain: -1, s1"/1 -> Math Function2/1
  "s1(2k), s1(2k+1)"/2 -> "gain: -1, s1"/1, "x1_ss1(n), unsorted"/2
  "s0(2k), s0(2k+1)"/1 -> Math Function3/1, "x0_ss1(n), unsorted"/1
  Math Function1/1 -> "x0_ss2(n), unsorted"/1
  "s1(2k), s1(2k+1)"/1 -> Math Function4/1, "x1_ss1(n), unsorted"/1
  Math Function3/1 -> "x0_ss2(n), unsorted"/2
  Math Function4/1 -> "x1_ss2(n), unsorted"/2
  "x0_ss1(n), unsorted"/1 -> x0_ss1(n)/1
  Math Function2/1 -> "x1_ss2(n), unsorted"/1
  "x0_ss2(n), unsorted"/1 -> x0_ss2(n)/1
  "x1_ss1(n), unsorted"/1 -> x1_ss1(n)/1
  "x1_ss2(n), unsorted"/1 -> x1_ss2(n)/1
  x0_ss1(n)/1 -> Switch1/4, Switch1/3
  x0_ss2(n)/1 -> Switch2/4, Switch2/3
  x1_ss1(n)/1 -> Switch3/4
  x1_ss2(n)/1 -> Switch4/4
  Switch1/1 -> "STBC, SS1"/2
  Switch2/1 -> "STBC, SS2"/2
  Switch3/1 -> "STBC, SS3"/2
  Switch4/1 -> "STBC, SS4"/2
  "STBC, SS1"/1 -> Add CS1/1
  "STBC, SS2"/1 -> Add CS2/1
  "STBC, SS3"/1 -> Add CS3/1
  "STBC, SS4"/1 -> Add CS4/1
  "CS, ss4"/1 -> Add CS4/2
  "CS, ss3"/1 -> Add CS3/2
  "CS, ss2"/1 -> Add CS2/2
  "CS, ss1"/1 -> Add CS1/2
  Add CS1/1 -> "out, SS1"/1
  Add CS2/1 -> "out, SS2"/1
  Add CS3/1 -> "out, SS3"/1
  Add CS4/1 -> "out, SS4"/1

== system ieee80211n/Select symbols ==
  In1 : Inport  Orientation=left  Port=1  LatchInput=off
  Select symbols : Selector  Orientation=left  InputType=Matrix  Elements=[39:64 1:27]  Rows=params.RXSelectFFTIndices  Columns=-1  InputPortWidth=64
  Out1 : Outport  Orientation=left
  wires:
  In1/1 -> Select symbols/1
  Select symbols/1 -> Out1/1

== system ieee80211n/Select symbols1 ==
  In1 : Inport  Orientation=left  Port=1  LatchInput=off
  Select symbols : Selector  Orientation=left  InputType=Matrix  Elements=[39:64 1:27]  Rows=params.RXSelectFFTIndices  Columns=-1  InputPortWidth=64
  Out1 : Outport  Orientation=left
  wires:
  In1/1 -> Select symbols/1
  Select symbols/1 -> Out1/1

== system ieee80211n/Select symbols2 ==
  In1 : Inport  Orientation=left  Port=1  LatchInput=off
  Select symbols : Selector  Orientation=left  InputType=Matrix  Elements=[39:64 1:27]  Rows=params.RXSelectFFTIndices  Columns=-1  InputPortWidth=64
  Out1 : Outport  Orientation=left
  wires:
  In1/1 -> Select symbols/1
  Select symbols/1 -> Out1/1

== system ieee80211n/Select symbols3 ==
  In1 : Inport  Orientation=left  Port=1  LatchInput=off
  Select symbols : Selector  Orientation=left  InputType=Matrix  Elements=[39:64 1:27]  Rows=params.RXSelectFFTIndices  Columns=-1  InputPortWidth=64
  Out1 : Outport  Orientation=left
  wires:
  In1/1 -> Select symbols/1
  Select symbols/1 -> Out1/1

== system ieee80211n/TGn channel model ==
  In SS1 : Inport  Orientation=down  Port=1  LatchInput=off
  In SS2 : Inport  Orientation=down  Port=2  LatchInput=off
  In SS3 : Inport  Orientation=down  Port=3  LatchInput=off
  In SS4 : Inport  Orientation=down  Port=4  LatchInput=off
  Ch Output Rx Streams : simulink/Math Operations/Reshape  Orientation=down  OutputDimensionality=Customize  OutputDimensions=[5*params.OFDMTotSymPerFrame*params.NFFT2, 4]
  Counter : dspswit3/Counter  Orientation=left  Direction=Up  CountEvent=Free running  CounterSize=32 bits  MaxCount=255  InitialCount=0  Output=Count  HitValue=32  ResetInput=off  SamplesPerFrame=1  Ts=params.minBitPeriod*(params.NSS*params.maxBitsPerBlock)  CntDtype=double  HitDtype=Logical
  FIR Decimation : dspmlti3/FIR Decimation  Orientation=down  DialogController=dspDDGCreate  DialogControllerArgs=DataTag35  h=5*fir1(25,1/4.5) %fir1(35,0.5*2/5)  D=5  framing=Maintain input frame rate  outputBufInitCond=0  roundingMode=Floor  overflowMode=off
  FIR Decimation1 : dspmlti3/FIR Decimation  Orientation=down  DialogController=dspDDGCreate  DialogControllerArgs=DataTag36  h=5*fir1(25,1/4.5) %fir1(35,0.5*2/5)  D=5  framing=Maintain input frame rate  outputBufInitCond=0  roundingMode=Floor  overflowMode=off
  FIR Decimation2 : dspmlti3/FIR Decimation  Orientation=down  DialogController=dspDDGCreate  DialogControllerArgs=DataTag37  h=5*fir1(25,1/4.5) %fir1(35,0.5*2/5)  D=5  framing=Maintain input frame rate  outputBufInitCond=0  roundingMode=Floor  overflowMode=off
  FIR Decimation3 : dspmlti3/FIR Decimation  Orientation=down  DialogController=dspDDGCreate  DialogControllerArgs=DataTag38  h=5*fir1(25,1/4.5) %fir1(35,0.5*2/5)  D=5  framing=Maintain input frame rate  outputBufInitCond=0  roundingMode=Floor  overflowMode=off
  FIR Interpolation : dspmlti3/FIR Interpolation  Orientation=down  DialogController=dspDDGCreate  DialogControllerArgs=DataTag39  h=0.955*fir1(25,1/4)  L=5  framing=Maintain input frame rate  outputBufInitCond=0  roundingMode=Floor  overflowMode=off
  FIR Interpolation1 : dspmlti3/FIR Interpolation  Orientation=down  DialogController=dspDDGCreate  DialogControllerArgs=DataTag40  h=0.955*fir1(25,1/4)  L=5  framing=Maintain input frame rate  outputBufInitCond=0  roundingMode=Floor  overflowMode=off
  FIR Interpolation2 : dspmlti3/FIR Interpolation  Orientation=down  DialogController=dspDDGCreate  DialogControllerArgs=DataTag41  h=0.955*fir1(25,1/4)  L=5  framing=Maintain input frame rate  outputBufInitCond=0  roundingMode=Floor  overflowMode=off
  FIR Interpolation3 : dspmlti3/FIR Interpolation  Orientation=down  DialogController=dspDDGCreate  DialogControllerArgs=DataTag42  h=0.955*fir1(25,1/4)  L=5  framing=Maintain input frame rate  outputBufInitCond=0  roundingMode=Floor  overflowMode=off
  Nltf : Constant  Orientation=left  Value=params.NLTF
  Nrx : Constant  Orientation=left  Value=params.NRX
  Ntx : Constant  Orientation=left  Value=params.NTX
  Rx streams : S-Function  Orientation=down  AncestorBlock=dspindex/Multiport Selector  FunctionName=sdspmultiportsel  Parameters=rowsOrCols, numOutports, flatIdxVect, flatLenVect, idxErrMode  mask(Multiport Selector){rowsOrCols=Columns, idxCellArray={1 2 3 4}, idxErrMode=Clip Index}
      mask prompts: rowsOrCols "Select:"; idxCellArray "Indices to output:"; idxErrMode "Invalid index:"
      mask help: Output specified rows or columns to one or more output ports. The number of output ports is determined by the number of index vectors, each specified as a separate vector entry in a cell array. Indices are 1-based and need not be unique.
      mask init:
      | [numOutports, flatLenVect, flatIdxVect] = dspblkmultiportsel(idxCellArray);
      mask Help: web(dspbhelp);
      mask StyleString: popup(Rows|Columns),edit,popup(Clip Index|Clip and Warn|Generate Error)
      mask Display: disp(['Select\n' &1]);
  TGn Channel Inputs : simulink/Math Operations/Matrix Concatenation  Orientation=down  numInports=8  catMethod=Vertical
  TGn Channel Model : MATLABFcn  Orientation=down  MATLABFcn=ch_model  OutputDimensions=[5*4*params.OFDMTotSymPerFrame*params.NFFT2 1]  Output1D=off
  Out SS1 : Outport  Orientation=down
  Out SS2 : Outport  Orientation=down  Port=2
  Out SS3 : Outport  Orientation=down  Port=3
  Out SS4 : Outport  Orientation=down  Port=4
  wires:
  Rx streams/1 -> FIR Decimation1/1
  In SS1/1 -> FIR Interpolation1/1
  In SS2/1 -> FIR Interpolation2/1
  In SS3/1 -> FIR Interpolation3/1
  In SS4/1 -> FIR Interpolation/1
  Rx streams/2 -> FIR Decimation2/1
  Rx streams/3 -> FIR Decimation3/1
  Rx streams/4 -> FIR Decimation/1
  Counter/1 -> TGn Channel Inputs/1
  Ntx/1 -> TGn Channel Inputs/2
  Nrx/1 -> TGn Channel Inputs/3
  TGn Channel Inputs/1 -> TGn Channel Model/1
  Ch Output Rx Streams/1 -> Rx streams/1
  TGn Channel Model/1 -> Ch Output Rx Streams/1
  FIR Decimation/1 -> Out SS4/1
  FIR Decimation3/1 -> Out SS3/1
  FIR Decimation2/1 -> Out SS2/1
  FIR Decimation1/1 -> Out SS1/1
  FIR Interpolation/1 -> TGn Channel Inputs/8
  FIR Interpolation3/1 -> TGn Channel Inputs/7
  FIR Interpolation2/1 -> TGn Channel Inputs/6
  FIR Interpolation1/1 -> TGn Channel Inputs/5
  Nltf/1 -> TGn Channel Inputs/4

== system ieee80211n/Transform to frequency domain ==
  in : Inport  Port=1  LatchInput=off
  FFT : dspxfrm3/FFT  DialogController=dspDDGCreate  DialogControllerArgs=DataTag43  CompMethod=Table lookup  TableOpt=Speed  BitRevOrder=off  SkipNorm=on  roundingMode=Floor  overflowMode=off
  Frame Status Conversion : dspsigattribs/Frame Status Conversion  growRefPort=off  outframe=Frame-based
  Normalize : Gain  Gain=sqrt(params.NST)/params.NFFT  SaturateOnIntegerOverflow=on
  out : Outport
  wires:
  FFT/1 -> Normalize/1
  Normalize/1 -> Frame Status Conversion/1
  in/1 -> FFT/1
  Frame Status Conversion/1 -> out/1

== system ieee80211n/Transform to frequency domain1 ==
  in : Inport  Port=1  LatchInput=off
  FFT : dspxfrm3/FFT  DialogController=dspDDGCreate  DialogControllerArgs=DataTag44  CompMethod=Table lookup  TableOpt=Speed  BitRevOrder=off  SkipNorm=on  roundingMode=Floor  overflowMode=off
  Frame Status Conversion : dspsigattribs/Frame Status Conversion  growRefPort=off  outframe=Frame-based
  Normalize : Gain  Gain=sqrt(params.NST)/params.NFFT  SaturateOnIntegerOverflow=on
  out : Outport
  wires:
  FFT/1 -> Normalize/1
  Normalize/1 -> Frame Status Conversion/1
  in/1 -> FFT/1
  Frame Status Conversion/1 -> out/1

== system ieee80211n/Transform to frequency domain2 ==
  in : Inport  Port=1  LatchInput=off
  FFT : dspxfrm3/FFT  DialogController=dspDDGCreate  DialogControllerArgs=DataTag45  CompMethod=Table lookup  TableOpt=Speed  BitRevOrder=off  SkipNorm=on  roundingMode=Floor  overflowMode=off
  Frame Status Conversion : dspsigattribs/Frame Status Conversion  growRefPort=off  outframe=Frame-based
  Normalize : Gain  Gain=sqrt(params.NST)/params.NFFT  SaturateOnIntegerOverflow=on
  out : Outport
  wires:
  FFT/1 -> Normalize/1
  Normalize/1 -> Frame Status Conversion/1
  in/1 -> FFT/1
  Frame Status Conversion/1 -> out/1

== system ieee80211n/Transform to frequency domain3 ==
  in : Inport  Port=1  LatchInput=off
  FFT : dspxfrm3/FFT  DialogController=dspDDGCreate  DialogControllerArgs=DataTag46  CompMethod=Table lookup  TableOpt=Speed  BitRevOrder=off  SkipNorm=on  roundingMode=Floor  overflowMode=off
  Frame Status Conversion : dspsigattribs/Frame Status Conversion  growRefPort=off  outframe=Frame-based
  Normalize : Gain  Gain=sqrt(params.NST)/params.NFFT  SaturateOnIntegerOverflow=on
  out : Outport
  wires:
  FFT/1 -> Normalize/1
  Normalize/1 -> Frame Status Conversion/1
  in/1 -> FFT/1
  Frame Status Conversion/1 -> out/1

== system ieee80211n/Transform to time domain ==
  in : Inport  Port=1  LatchInput=off
  IFFT : dspxfrm3/IFFT  DialogController=dspDDGCreate  DialogControllerArgs=DataTag47  CompMethod=Table lookup  TableOpt=Speed  BitRevOrder=off  cs_in=off  SkipNorm=off  mode=Complex  roundingMode=Floor  overflowMode=off
  Normalize : Gain  Gain=params.NFFT/sqrt(params.NST)  SaturateOnIntegerOverflow=on
  Shift for FFT : Selector  InputType=Matrix  Elements=[27:64 1:26]  Rows=params.TXFFTShiftIndices  Columns=-1  InputPortWidth=64
  Zero Pad : dspsigops/Zero Pad  padSigAt=End  zpadAlong=Columns  padNumOutRowsSpecMethod=User-specified  numOutRows=params.NFFT  padNumOutColsSpecMethod=User-specified  numOutCols=1  trunc_flag=None
  out : Outport
  wires:
  in/1 -> Zero Pad/1
  IFFT/1 -> Normalize/1
  Normalize/1 -> out/1
  Zero Pad/1 -> Shift for FFT/1
  Shift for FFT/1 -> IFFT/1

== system ieee80211n/Transform to time domain1 ==
  in : Inport  Port=1  LatchInput=off
  IFFT : dspxfrm3/IFFT  DialogController=dspDDGCreate  DialogControllerArgs=DataTag48  CompMethod=Table lookup  TableOpt=Speed  BitRevOrder=off  cs_in=off  SkipNorm=off  mode=Complex  roundingMode=Floor  overflowMode=off
  Normalize : Gain  Gain=params.NFFT/sqrt(params.NST)  SaturateOnIntegerOverflow=on
  Shift for FFT : Selector  InputType=Matrix  Elements=[27:64 1:26]  Rows=params.TXFFTShiftIndices  Columns=-1  InputPortWidth=64
  Zero Pad : dspsigops/Zero Pad  padSigAt=End  zpadAlong=Columns  padNumOutRowsSpecMethod=User-specified  numOutRows=params.NFFT  padNumOutColsSpecMethod=User-specified  numOutCols=1  trunc_flag=None
  out : Outport
  wires:
  in/1 -> Zero Pad/1
  IFFT/1 -> Normalize/1
  Normalize/1 -> out/1
  Zero Pad/1 -> Shift for FFT/1
  Shift for FFT/1 -> IFFT/1

== system ieee80211n/Transform to time domain2 ==
  in : Inport  Port=1  LatchInput=off
  IFFT : dspxfrm3/IFFT  DialogController=dspDDGCreate  DialogControllerArgs=DataTag49  CompMethod=Table lookup  TableOpt=Speed  BitRevOrder=off  cs_in=off  SkipNorm=off  mode=Complex  roundingMode=Floor  overflowMode=off
  Normalize : Gain  Gain=params.NFFT/sqrt(params.NST)  SaturateOnIntegerOverflow=on
  Shift for FFT : Selector  InputType=Matrix  Elements=[27:64 1:26]  Rows=params.TXFFTShiftIndices  Columns=-1  InputPortWidth=64
  Zero Pad : dspsigops/Zero Pad  padSigAt=End  zpadAlong=Columns  padNumOutRowsSpecMethod=User-specified  numOutRows=params.NFFT  padNumOutColsSpecMethod=User-specified  numOutCols=1  trunc_flag=None
  out : Outport
  wires:
  in/1 -> Zero Pad/1
  IFFT/1 -> Normalize/1
  Normalize/1 -> out/1
  Zero Pad/1 -> Shift for FFT/1
  Shift for FFT/1 -> IFFT/1

== system ieee80211n/Transform to time domain3 ==
  in : Inport  Port=1  LatchInput=off
  IFFT : dspxfrm3/IFFT  DialogController=dspDDGCreate  DialogControllerArgs=DataTag50  CompMethod=Table lookup  TableOpt=Speed  BitRevOrder=off  cs_in=off  SkipNorm=off  mode=Complex  roundingMode=Floor  overflowMode=off
  Normalize : Gain  Gain=params.NFFT/sqrt(params.NST)  SaturateOnIntegerOverflow=on
  Shift for FFT : Selector  InputType=Matrix  Elements=[27:64 1:26]  Rows=params.TXFFTShiftIndices  Columns=-1  InputPortWidth=64
  Zero Pad : dspsigops/Zero Pad  padSigAt=End  zpadAlong=Columns  padNumOutRowsSpecMethod=User-specified  numOutRows=params.NFFT  padNumOutColsSpecMethod=User-specified  numOutCols=1  trunc_flag=None
  out : Outport
  wires:
  in/1 -> Zero Pad/1
  IFFT/1 -> Normalize/1
  Normalize/1 -> out/1
  Zero Pad/1 -> Shift for FFT/1
  Shift for FFT/1 -> IFFT/1

== system ieee80211n/adjust settings ==
  note: This subsystem is empty.
      | It is used for setting parameter values (in the mask).

== system ieee80211n/adjust settings2 ==
  note: This subsystem is empty.
      | It is used for setting parameter values (in the mask).

== system ieee80211n/cyclic prefix ==
  in : Inport  Port=1  LatchInput=off
  Add Cyclic Prefix : Selector  InputType=Matrix  Elements=[49:64 1:64]  Rows=params.TXCyclicPrefixIndices  Columns=-1  InputPortWidth=64
  "Cyclic shift, SS1" : Subsystem
      mask Display: disp('Cyclic Shift\nDelay')
  out : Outport
  wires:
  Add Cyclic Prefix/1 -> out/1
  in/1 -> "Cyclic shift, SS1"/1(in)
  "Cyclic shift, SS1"/1(out) -> Add Cyclic Prefix/1
